simulink model "qx2"  (R2023b)
settings: Solver=FixedStepAuto  StartTime=0.0  StopTime=200  FixedStep=0.01  RelTol=1e-3
undefined symbols (not defined in the file or in its folder): w2
settings Model: Creator=asus  LastModifiedBy=asus

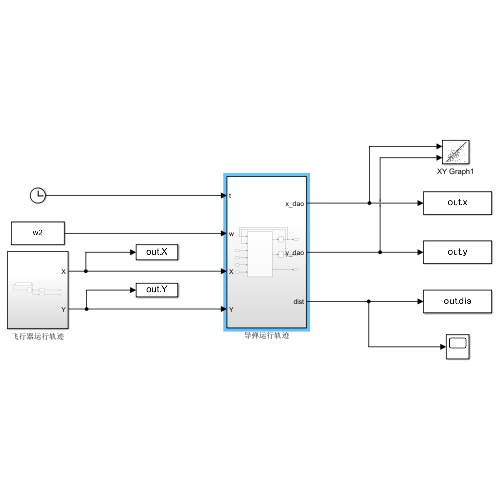
[thumbnail: Simulink's stored preview of the top-level diagram]
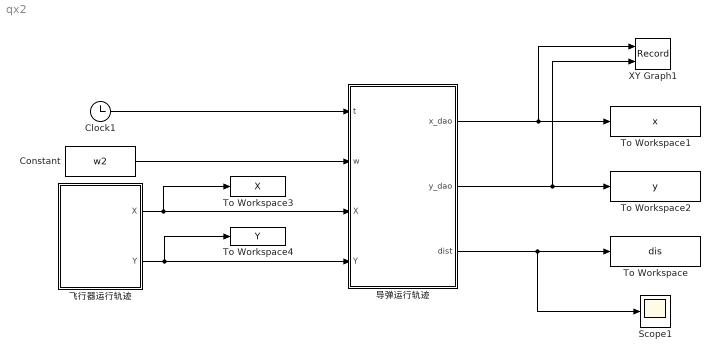
== system qx2 ==
  Clock1 : Clock
  Constant : Constant  Value=w2
  Scope1 : Scope
  To Workspace : ToWorkspace  VariableName=dis  SaveFormat=Timeseries  SampleTime=-1
  To Workspace1 : ToWorkspace  VariableName=x  SaveFormat=Timeseries  SampleTime=-1
  To Workspace2 : ToWorkspace  VariableName=y  SaveFormat=Timeseries  SampleTime=-1
  To Workspace3 : ToWorkspace  VariableName=X  SaveFormat=Timeseries  SampleTime=-1
  To Workspace4 : ToWorkspace  VariableName=Y  SaveFormat=Timeseries  SampleTime=-1
  XY Graph1 : Record  FileSettingsInternal="{\"entries\":[{\"content\":{\"excelSettings\":{\"content\":{},\"type\":\"Streamout.ExcelSettings\"}},\"type\":\"Streamout.FileSettingStorage\",\"uuid\":\"\"}],\"packageUris\":[\"http:\\/\\/schema.mathworks.com\\/mf0\\/streamout_blocks\\/R2020a\"],\"version\":\"1.0\"}"  Layout=[1 1]  SignalsInternal="{\"entries\":[{\"content\":{\"signals\":[{\"content\":{\"blockPath\":[],\"dimensions\":[1],\"domain\":\"\",\"lineColor\":\"#a2142f\",\"plots\":[1],\"port\":1,\"sid\":[\"\"],\"signalID\":51729,\"signalName\":\"导弹运行轨迹:1\"},\"type\":\"RecordBlkView.Signal\",\"uuid\":\"\"},{\"content\":{\"blockPath\":[],\"dimensions\":[1],\"domain\":\"\",\"lineColor\":\"#139fff\",\"plots\":[1],\"port\":2,\"sid\":[\"\"],\"signalID\":51733,\"signalName\":\"导弹运行轨迹:2\"},\"type\":\"RecordBlkView.Signal\",\"uuid\":\"\"}]},\"type\":\"RecordBlkView.InputSignals\",\"uuid\":\"\"}],\"packageUris\":[\"http:\\/\\/schema.mathworks.com\\/mf0\\/streamout_blocks\\/R2020a\"],\"version\":\"1.0\"}"  VisualizationBindings="{\"xyplotplugin\":{\"info\":[{\"series\":[{\"bindingParametersList\":[{\"parameter\":\"X-Axis\",\"signalID\":51729,\"signalName\":\"导弹运行轨迹:1\"},{\"parameter\":\"Y-Axis\",\"signalID\":51733,\"signalName\":\"导弹运行轨迹:2\"}],\"seriesID\":56045}],\"subplotID\":1}]}}"  CompatibilityTag=XY
  导弹运行轨迹 : Subsystem
  飞行器运行轨迹 : Subsystem
  wires:
  飞行器运行轨迹/1(X) -> To Workspace3/1, 导弹运行轨迹/3(X)
  飞行器运行轨迹/2(Y) -> To Workspace4/1, 导弹运行轨迹/4(Y)
  导弹运行轨迹/3(dist) -> Scope1/1, To Workspace/1
  导弹运行轨迹/1(x_dao) -> XY Graph1/1, To Workspace1/1
  导弹运行轨迹/2(y_dao) -> To Workspace2/1, XY Graph1/2
  Clock1/1 -> 导弹运行轨迹/1(t)
  Constant/1 -> 导弹运行轨迹/2(w)

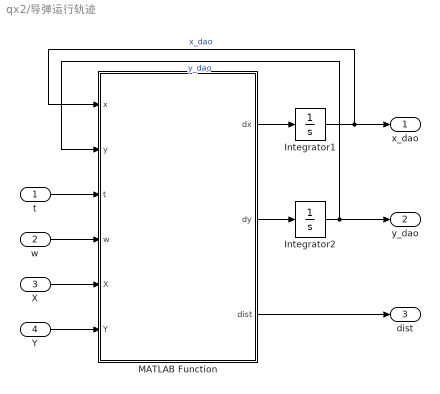
== system qx2/导弹运行轨迹 ==
  t : Inport
  w : Inport  Port=2
  X : Inport  Port=3
  Y : Inport  Port=4
  Integrator1 : Integrator
  Integrator2 : Integrator
  MATLAB Function : MATLAB Function  TreatAsAtomicUnit=on
  x_dao : Outport
  y_dao : Outport  Port=2
  dist : Outport  Port=3
  wires:
  Y/1 -> MATLAB Function/6(Y)
  Integrator1/1 -> x_dao/1, MATLAB Function/1(x)  "x_dao"
  MATLAB Function/1(dx) -> Integrator1/1
  MATLAB Function/3(dist) -> dist/1
  X/1 -> MATLAB Function/5(X)
  Integrator2/1 -> y_dao/1, MATLAB Function/2(y)  "y_dao"
  MATLAB Function/2(dy) -> Integrator2/1
  t/1 -> MATLAB Function/3(t)
  w/1 -> MATLAB Function/4(w)

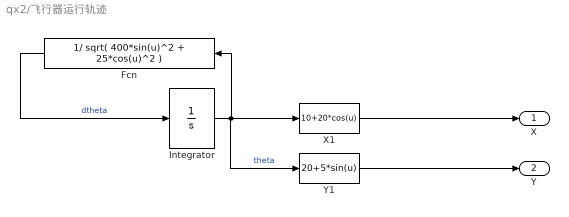
== system qx2/飞行器运行轨迹 ==
  Fcn : Fcn  Expr=1/ sqrt( 400*sin(u)^2 + 25*cos(u)^2 )
  Integrator : Integrator
  X1 : Fcn  Expr=10+20*cos(u)
  Y1 : Fcn  Expr=20+5*sin(u)
  X : Outport
  Y : Outport  Port=2
  wires:
  Integrator/1 -> Y1/1, X1/1, Fcn/1  "theta"
  Fcn/1 -> Integrator/1  "dtheta"
  Y1/1 -> Y/1
  X1/1 -> X/1

== matlab function qx2/导弹运行轨迹/MATLAB Function ==
  data: x input; dx output; y input; t input; dy output; dist output; w input; X input; Y input
function [dx,dy,dist] = fcn(x,y,t,w,X,Y)
x_fei = X;
y_fei = Y;
dist = sqrt( (x_fei - x)^2 + (y_fei - y)^2 );
dx = w * (x_fei - x) / dist;
dy = w * (y_fei - y) / dist;
